simulink model "Algorithm_to_deploy"  (R2025b)
settings: Solver=ode4  StartTime=0.0  StopTime=Tfin  FixedStep=0.005  RelTol=1e-3  EnableMultiTasking=on
undefined symbols (not defined in the file): A_zeta_f, A_zeta_tau, C_zeta_f, C_zeta_tau, eigs_NDO_force, eigs_NDO_torque, F1, F2, inertia_factor, J, m, mass_factor, NDOB_force, NDOB_torque, Ts_hw
settings Model: Creator=baldo  LastModifiedBy=robyd
settings DataIOCC: SaveOutput=off  SaveTime=off
settings OptimizationCC: DefaultParameterBehavior=Inlined  EnhancedBackFolding=on  PassReuseOutputArgsAs=Individual arguments  ZeroExternalMemoryAtStartup=off  ZeroInternalMemoryAtStartup=off  MaxStackSize=512  OptimizeBlockOrder=speed  DifferentSizesBufferReuse=on  OptimizationCustomize=off  EfficientTunableParamExpr=on
settings DebuggingCC: ParameterTunabilityLossMsg=error  UnconnectedInputMsg=warning  UnconnectedOutputMsg=warning  UnconnectedLineMsg=warning
settings HardwareCC: ProdBitPerPointer=32.0  ProdBitPerSizeT=32.0  ProdBitPerPtrDiffT=32.0  ProdLargestAtomicInteger=Long  ProdLargestAtomicFloat=Double  ProdWordSize=32.0  ProdLongLongMode=on  ProdHWDeviceType=ARM Compatible->ARM Cortex-M
settings ModelReferenceCC: EnableRefExpFcnMdlSchedulingChecks=on  PropagateVarSize=During execution
settings SFSimCC: MATLABDynamicMemAlloc=off
settings RTWCC: SystemTargetFile=ert.tlc  HardwareBoard=STM32H7xx Based (Single-core)  TemplateMakefile=ert_default_tmf  Toolchain=GNU Tools for ARM Embedded Processors  CodeExecutionProfiling=on  GPUComputeCapability=3.5  DLArmComputeVersion=19.05  Description=Embedded Coder
settings CodeAppCC: ForceParamTrailComments=on  IgnoreCustomStorageClasses=off  OperatorAnnotations=on  SimulinkDataObjDesc=on  SFDataObjDesc=on  InsertBlockDesc=on
settings ERTTargetCC: ExtModeTransport=3.0  ExtModeStaticAlloc=on  ExtModeStaticAllocSize=2048.0  ExtModeMexFile=ext_xcp  ExtModeIntrfLevel=Level2 - Open  TargetLangStandard=C99 (ISO)  CodeReplacementLibrary=ARM Cortex-M  SupportVariableSizeSignals=on

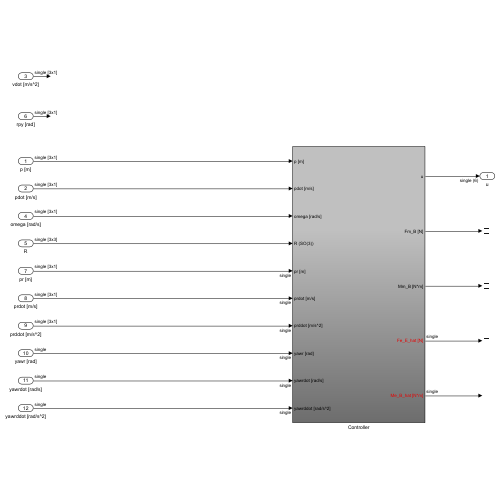
[thumbnail: Simulink's stored preview of the top-level diagram]
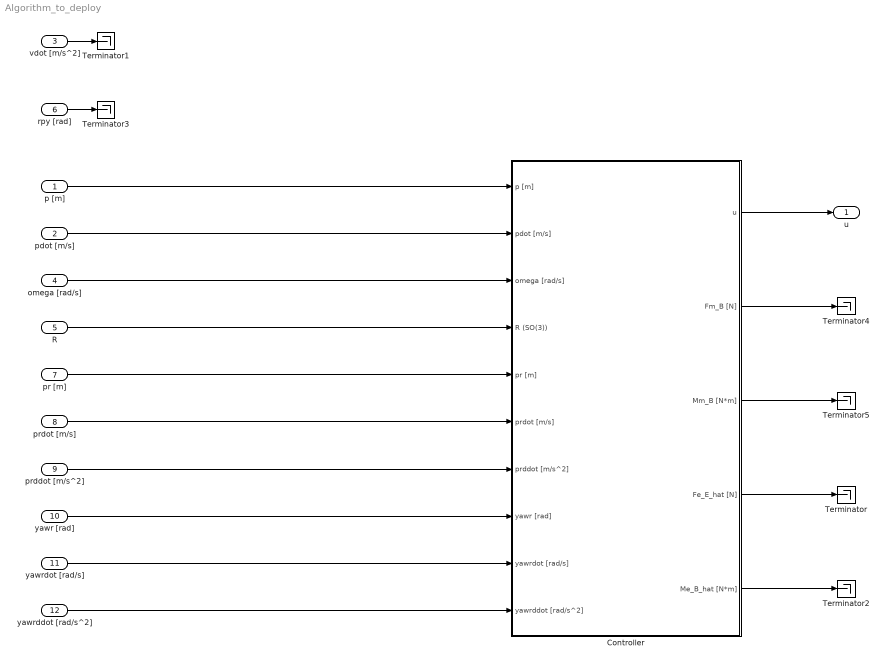
== system Algorithm_to_deploy ==
  p [m] : Inport  OutDataTypeStr=single  PortDimensions=[3 1]  SampleTime=[0.0050000000000000001,0]
  pdot [m/s] : Inport  Port=2  OutDataTypeStr=single  PortDimensions=[3 1]  SampleTime=[0.0050000000000000001,0]
  vdot [m/s^2] : Inport  Port=3  OutDataTypeStr=single  PortDimensions=[3 1]  SampleTime=[0.0050000000000000001,0]
  omega [rad/s] : Inport  Port=4  OutDataTypeStr=single  PortDimensions=[3 1]  SampleTime=[0.0050000000000000001,0]
  R : Inport  Port=5  OutDataTypeStr=single  PortDimensions=[3 3]  SampleTime=[0.0050000000000000001,0]
  rpy [rad] : Inport  Port=6  OutDataTypeStr=single  PortDimensions=[3 1]  SampleTime=[0.0050000000000000001,0]
  pr [m] : Inport  Port=7  OutDataTypeStr=single  PortDimensions=[3 1]  SampleTime=[0.0050000000000000001,0]
  prdot [m/s] : Inport  Port=8  OutDataTypeStr=single  PortDimensions=[3 1]  SampleTime=[0.0050000000000000001,0]
  prddot [m/s^2] : Inport  Port=9  OutDataTypeStr=single  PortDimensions=[3 1]  SampleTime=[0.0050000000000000001,0]
  yawr [rad] : Inport  Port=10  OutDataTypeStr=single  PortDimensions=1  SampleTime=[0.0050000000000000001,0]
  yawrdot [rad/s] : Inport  Port=11  OutDataTypeStr=single  PortDimensions=1  SampleTime=[0.0050000000000000001,0]
  yawrddot [rad/s^2] : Inport  Port=12  OutDataTypeStr=single  PortDimensions=1  SampleTime=[0.0050000000000000001,0]
  Controller : Subsystem
  Terminator{,1..5} (6 alike) : Terminator
  u : Outport  OutDataTypeStr=single  PortDimensions=6  SampleTime=[0.0050000000000000001,0]
  wires:
  vdot [m/s^2]/1 -> Terminator1/1
  rpy [rad]/1 -> Terminator3/1
  p [m]/1 -> Controller/1(p [m])
  pdot [m/s]/1 -> Controller/2(pdot [m/s])
  omega [rad/s]/1 -> Controller/3(omega [rad/s])
  R/1 -> Controller/4(R (SO(3)))
  pr [m]/1 -> Controller/5(pr [m])
  prdot [m/s]/1 -> Controller/6(prdot [m/s])
  prddot [m/s^2]/1 -> Controller/7(prddot [m/s^2])
  yawr [rad]/1 -> Controller/8(yawr [rad])
  yawrdot [rad/s]/1 -> Controller/9(yawrdot [rad/s])
  yawrddot [rad/s^2]/1 -> Controller/10(yawrddot [rad/s^2])
  Controller/1(u) -> u/1
  Controller/2(Fm_B [N]) -> Terminator4/1
  Controller/3(Mm_B [N*m]) -> Terminator5/1
  Controller/4(Fe_E_hat [N]) -> Terminator/1
  Controller/5(Me_B_hat [N*m]) -> Terminator2/1

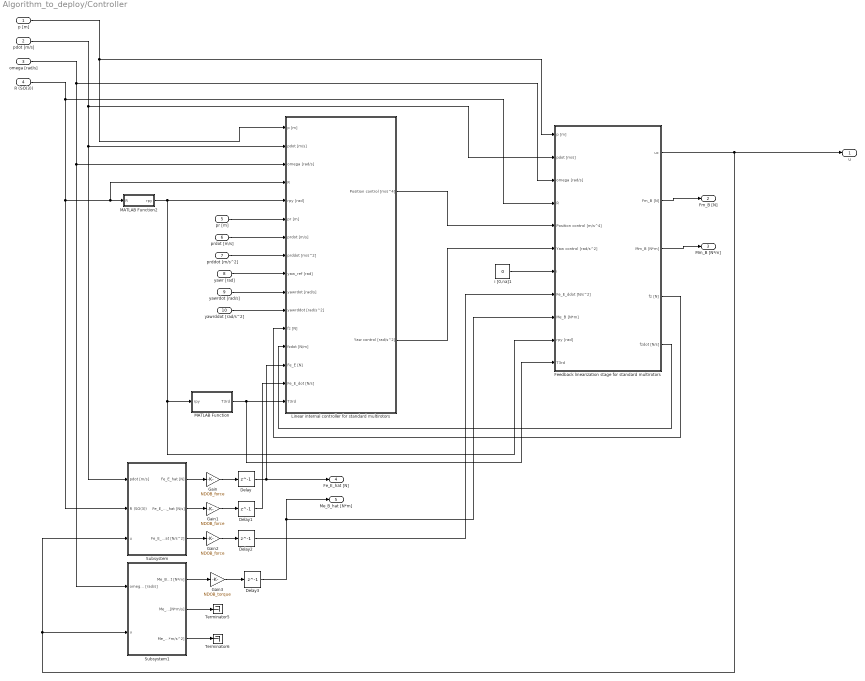
== system Algorithm_to_deploy/Controller ==
  p [m] : Inport
  pdot [m/s] : Inport  Port=2
  omega [rad/s] : Inport  Port=3
  R (SO(3)) : Inport  Port=4
  pr [m] : Inport  Port=5  OutDataTypeStr=single
  prdot [m/s] : Inport  Port=6  OutDataTypeStr=single
  prddot [m/s^2] : Inport  Port=7  OutDataTypeStr=single
  yawr [rad] : Inport  Port=8  OutDataTypeStr=single
  yawrdot [rad/s] : Inport  Port=9  OutDataTypeStr=single
  yawrddot [rad/s^2] : Inport  Port=10  OutDataTypeStr=single
  Delay{,1..3} (4 alike) : Delay  DelayLength=1  InitialCondition=0
  Feedback linearization stage for standard multirotors : Subsystem  mask{mask_m=single(m*mass_factor), mask_J=single(J*inertia_factor), mask_rg_B=zeros(3,1), mask_F1=single(F1), mask_F2=single(F2), mask_thrustmax=1, mask_fz0=single(m*9.8), mask_Ts=Ts_hw}
      mask prompts: mask_m "Mass [kg]"; mask_J "Inertia Tensor [kg*m^2]"; mask_rg_B "Center of mass [m]"; mask_F1 "Control force input matrix"; mask_F2 "Control moment input matrix"; mask_thrustmax "Max thrust [N]"; mask_fz0 "Upward lift force"; mask_Ts "Sample time"
      mask init:
      | % Wrappers
      |     e1 = single([1; 0; 0]);
      |     e2 = single([0; 1; 0]);
      |     e3 = single([0; 0; 1]);
      |     
      |     %%%%%%%%%%%%%%%%%%%%%%%%%%%%%%%%%%%%%%%%%%%%
      |     %    Some general paramater
      |     %%%%%%%%%%%%%%%%%%%%%%%%%%%%%%%%%%%%%%%%%%%%
      |     mask_Jinv = inv(mask_J);
      |     mask_g = single(9.8);
      |     mask_na = size(mask_F1,2);
      | 
      |     %%%%%%%%%%%%%%%%%%%%%%%%%%%%%%%%%%%%%%%%%%%%
      |     %    Allocation for standard multirotors
      |     %%%%%%%%%%%%%%%%%%%%%%%%%%%%%%%%%%%%%%%%%%%%
      |     A = [mask_F1(3,:); mask_F2];
      |     A_pinv = single(pinv(A));
      mask DialogControl DescGroupVar Prompt: Feedback linearization stage for standard multirotors
      mask DialogControl DescTextVar Prompt: Dynamic feedback linearization for standard multirotors. Moore-Penrose allocation. The dynamic estension is "exact".
      mask DialogControl Control3 Prompt: Author: Alessandro Baldini
      mask DialogControl ParameterGroupVar Prompt: Multirotor parameters
      mask DialogControl Container4 Prompt: Initial condition and others
  Gain : Gain  Gain=NDOB_force
  Gain1 : Gain  Gain=NDOB_force
  Gain2 : Gain  Gain=NDOB_force
  Gain3 : Gain  Gain=NDOB_torque
  Linear internal controller for standard multirotors : Subsystem  mask{mask_m=single(m*mass_factor), mask_J=single(J*inertia_factor), mask_rg_B=zeros(3,1), mask_F1=single(F1), mask_F2=single(F2), mask_thrustmax=1, mask_xpoles=single([-3.0 -3.1 -3.2 -3.2 -1.3]/1.3), mask_ypoles=single([-3.0 -3.1 -3.2 -3.2 -1.3]/1.3), mask_zpoles=single([-3.0 -3.1 -3.2 -3.2 -1.3]/1.3), mask_yawpoles=single([-1 -2]), mask_chkPID=off, mask_chkYaw=off, mask_fz0=single(m*9.8), mask_Ts=Ts_hw}
      mask prompts: mask_m "Mass [kg]"; mask_J "Inertia Tensor [kg*m^2]"; mask_rg_B "Center of mass [m]"; mask_F1 "Control force input matrix"; mask_F2 "Control moment input matrix"; mask_thrustmax "Max thrust [N]"; mask_xpoles "Closed loop x poles"; mask_ypoles "Closed loop y poles"; mask_zpoles "Closed loop z poles"; mask_yawpoles "Closed loop yaw poles"; mask_chkPID "Enable position integrators"; mask_chkYaw "Enable yaw integrator"; mask_fz0 "Upward lift force"; mask_Ts "Sample time"
      mask init:
      | % Wrappers
      |     e1 = [1; 0; 0];
      |     e2 = [0; 1; 0];
      |     e3 = [0; 0; 1];
      |     
      |     %%%%%%%%%%%%%%%%%%%%%%%%%%%%%%%%%%%%%%%%%%%%
      |     %    Some general paramater
      |     %%%%%%%%%%%%%%%%%%%%%%%%%%%%%%%%%%%%%%%%%%%%
      |     mask_Jinv = inv(mask_J);
      |     mask_g = 9.8;
      |     mask_na = size(mask_F1,2);
      |     
      |     %%%%%%%%%%%%%%%%%%%%%%%%%%%%%%%%%%%%%%%%%%%%
      |     %    ( Control paramaters)
      |     %%%%%%%%%%%%%%%%%%%%%%%%%%%%%%%%%%%%%%%%%%%%
      |     % Calculation of outer loop parameters
      |     polyx = poly(mask_xpoles);
      |     polyy = poly(mask_ypoles);
      |     polyz = poly(mask_zpoles);
      |     polyyaw = poly(mask_yawpoles);
      | 
      |     if mask_chkPID == 1
      |         % Raw pole placement (with integral action)
      |         % We consider the first 5 poles (2 for yaw)
      |         mask_xpoles = mask_xpoles(1:5);
      |         mask_ypoles = mask_ypoles(1:5);
      |         mask_zpoles = mask_zpoles(1:5);
      |         polyyaw = polyyaw(1:2);
      | 
      |         polyx = poly(mask_xpoles);
      |         polyy = poly(mask_ypoles);
      |         polyz = poly(mask_zpoles);
      |         polyyaw = poly(mask_yawpoles);
      | 
      |         mask_k0 = diag([polyx(6) polyy(6) polyz(6)]);
      |         mask_k1 = diag([polyx(5) polyy(5) polyz(5)]);
      |         mask_k2 = diag([polyx(4) polyy(4) polyz(4)]);
      |         mask_k3 = diag([polyx(3) polyy(3) polyz(3)]);
      |         mask_k4 = diag([polyx(2) polyy(2) polyz(2)]);
      |         
      |         k0yaw = polyyaw(3);
      |         k1yaw = polyyaw(2);
      | 
      |     else
      |         % Raw pole placement (no integral action)
      |         % We consider the first 4 poles (2 for yaw)
      |         mask_xpoles = mask_xpoles(1:4);
      |         mask_ypoles = mask_ypoles(1:4);
      |         mask_zpoles = mask_zpoles(1:4);
      |         polyyaw = polyyaw(1:2);
      | 
      |         polyx = poly(mask_xpoles);
      |         polyy = poly(mask_ypoles);
      |         polyz = poly(mask_zpoles);
      |         polyyaw = poly(mask_yawpoles);
      | 
      |         mask_k0 = diag([polyx(5) polyy(5) polyz(5)]);
      |         mask_k1 = diag([polyx(4) polyy(4) polyz(4)]);
      |         mask_k2 = diag([polyx(3) polyy(3) polyz(3)]);
      |         mask_k3 = diag([polyx(2) polyy(2) polyz(2)]);
      |         mask_k4 = zeros(1,3); % Not used in this control mode
      | 
      |         k0yaw = polyyaw(3);
      |         k1yaw = polyyaw(2);
      |     end
      mask DialogControl DescGroupVar Prompt: Linear controller for standard multirotors
      mask DialogControl DescTextVar Prompt: Linear state space pole placement to couple with a feedback linearization stage. For standard multirotors.
      mask DialogControl Control3 Prompt: Author: Alessandro Baldini
      mask DialogControl ParameterGroupVar Prompt: Multirotor parameters
      mask DialogControl Container3 Prompt: Control paramaters (+1 pole each in case of integrators)
      mask DialogControl Container4 Prompt: Initial condition and others
  MATLAB Function : MATLAB Function  TreatAsAtomicUnit=on
  MATLAB Function2 : MATLAB Function  TreatAsAtomicUnit=on
  Subsystem : Subsystem  mask{mask_m=single(m*mass_factor), mask_F1=single(F1), mask_C=single(C_zeta_f), mask_A=single(A_zeta_f), mask_poles=single(eigs_NDO_force), mask_Ts=Ts_hw}
      mask prompts: mask_m "Mass [kg]"; mask_F1 "Control force input matrix"; mask_C "Exogenous system output matrix C"; mask_A "Exogenous system dynamics matrix A"; mask_poles "Poles to place"; mask_Ts "Sample time"
      mask init:
      | mask_nzeta = size(mask_A,2);
      |     if length(mask_poles) < mask_nzeta
      |         error(num2str(mask_nzeta) + " poles should be specified for the force estimation.")
      |     end
      | 
      |     mask_H = place(mask_A',mask_C',mask_poles(1:mask_nzeta))';
      |     mask_AH = mask_A - mask_H*mask_C;
      |     mask_g = 9.8;
      mask DialogControl DescGroupVar Prompt: Rigid body force observer - v 0.1
      mask DialogControl DescTextVar Prompt: Force observer for a rigid body through a Nonlinear Disturbance Observer (NDO), i.e., reduced order functional observer.
      mask DialogControl Control2 Prompt: Author: Alessandro Baldini
      mask DialogControl Mask_marameters Prompt: Parameters
      mask DialogControl Container3 Prompt: Initial conditions and others
  Subsystem1 : Subsystem  mask{mask_J=single(J*inertia_factor), mask_F2=single(F2), mask_C=single(C_zeta_tau), mask_A=single(A_zeta_tau), mask_poles=single(eigs_NDO_torque), mask_Ts=Ts_hw}
      mask prompts: mask_J "Inertia tensor [kg*m^2]"; mask_F2 "Control moment input matrix"; mask_C "Exogenous system output matrix C"; mask_A "Exogenous system dynamics matrix A"; mask_poles "Poles to place"; mask_Ts "Sample time"
      mask init:
      | mask_nzeta = size(mask_A,2);
      |     if length(mask_poles) < mask_nzeta
      |         error(num2str(mask_nzeta) + " poles should be specified for the torque estimation.")
      |     end
      | 
      |     mask_H = place(mask_A',mask_C',mask_poles(1:mask_nzeta))';
      |     mask_AH = mask_A - mask_H*mask_C;
      mask DialogControl DescGroupVar Prompt: Rigid body torque observer - v 0.1
      mask DialogControl DescTextVar Prompt: Torque observer for a rigid body through a Nonlinear Disturbance Observer (NDO), i.e., reduced order functional observer.
      mask DialogControl Control2 Prompt: Author: Alessandro Baldini
      mask DialogControl Mask_marameters Prompt: Parameters
      mask DialogControl Container3 Prompt: Initial conditions and others
  Terminator5 : Terminator
  Terminator6 : Terminator
  i [0,na]1 : Constant  Value=0  OutDataTypeStr=single  SampleTime=Ts_hw
  u : Outport
  Fm_B [N] : Outport  Port=2
  Mm_B [N*m] : Outport  Port=3
  Fe_E_hat [N] : Outport  Port=4  OutDataTypeStr=single
  Me_B_hat [N*m] : Outport  Port=5  OutDataTypeStr=single
  wires:
  i [0,na]1/1 -> Feedback linearization stage for standard multirotors/7(i)
  Gain3/1 -> Delay3/1
  Delay3/1 -> Feedback linearization stage for standard multirotors/9(Me_B [N*m]), Me_B_hat [N*m]/1
  Gain2/1 -> Delay2/1
  Subsystem1/2(Me_B_dot_hat [N*m/s]) -> Terminator5/1
  Feedback linearization stage for standard multirotors/3(Mm_B [N*m]) -> Mm_B [N*m]/1
  prddot [m/s^2]/1 -> Linear internal controller for standard multirotors/8(prddot [m/s^2])
  p [m]/1 -> Feedback linearization stage for standard multirotors/1(p [m]), Linear internal controller for standard multirotors/1(p [m])
  yawrddot [rad/s^2]/1 -> Linear internal controller for standard multirotors/11(yawrddot [rad/s^2])
  yawrdot [rad/s]/1 -> Linear internal controller for standard multirotors/10(yawrdot [rad/s])
  omega [rad/s]/1 -> Feedback linearization stage for standard multirotors/3(omega [rad/s]), Linear internal controller for standard multirotors/3(omega [rad/s]), Subsystem1/1(omega [rad/s])
  Subsystem1/1(Me_B_hat [N*m]) -> Gain3/1
  Linear internal controller for standard multirotors/1(" Position control [m/s^4]") -> Feedback linearization stage for standard multirotors/5(Position control [m/s^4])
  Gain1/1 -> Delay1/1
  Subsystem/1(Fe_E_hat [N]) -> Gain/1
  Subsystem/2(Fe_E_dot_hat [N/s]) -> Gain1/1
  Feedback linearization stage for standard multirotors/1(uc) -> Subsystem1/2(u), Subsystem/3(u), u/1
  Subsystem/3(Fe_E_ddot_hat [N/s^2]) -> Gain2/1
  Subsystem1/3(Me_B_ddot_hat [N*m/s^2]) -> Terminator6/1
  R (SO(3))/1 -> Subsystem/2(R (SO(3))), MATLAB Function2/1(R), Linear internal controller for standard multirotors/4(R), Feedback linearization stage for standard multirotors/4(R)
  Feedback linearization stage for standard multirotors/4(fz [N]) -> Linear internal controller for standard multirotors/12(fz [N])
  Feedback linearization stage for standard multirotors/5(fzdot [N/s]) -> Linear internal controller for standard multirotors/13(fzdot [N/m])
  prdot [m/s]/1 -> Linear internal controller for standard multirotors/7(prdot [m/s])
  Gain/1 -> Delay/1
  MATLAB Function2/1(rpy) -> MATLAB Function/1(rpy), Feedback linearization stage for standard multirotors/10(rpy [rad]), Linear internal controller for standard multirotors/5(rpy [rad])
  yawr [rad]/1 -> Linear internal controller for standard multirotors/9(yaw_ref [rad])
  Delay1/1 -> Linear internal controller for standard multirotors/15(Fe_E_dot [N/s])
  MATLAB Function/1(T3rd) -> Linear internal controller for standard multirotors/16(T3rd), Feedback linearization stage for standard multirotors/11(T3rd)
  Delay/1 -> Linear internal controller for standard multirotors/14(Fe_E [N]), Fe_E_hat [N]/1
  Delay2/1 -> Feedback linearization stage for standard multirotors/8(Fe_E_ddot [N/s^2])
  pdot [m/s]/1 -> Linear internal controller for standard multirotors/2(pdot [m/s]), Subsystem/1(pdot [m/s]), Feedback linearization stage for standard multirotors/2(pdot [m/s])
  Linear internal controller for standard multirotors/2(" Yaw control [rad/s^2]") -> Feedback linearization stage for standard multirotors/6(Yaw control [rad/s^2])
  pr [m]/1 -> Linear internal controller for standard multirotors/6(pr [m])
  Feedback linearization stage for standard multirotors/2(Fm_B [N]) -> Fm_B [N]/1

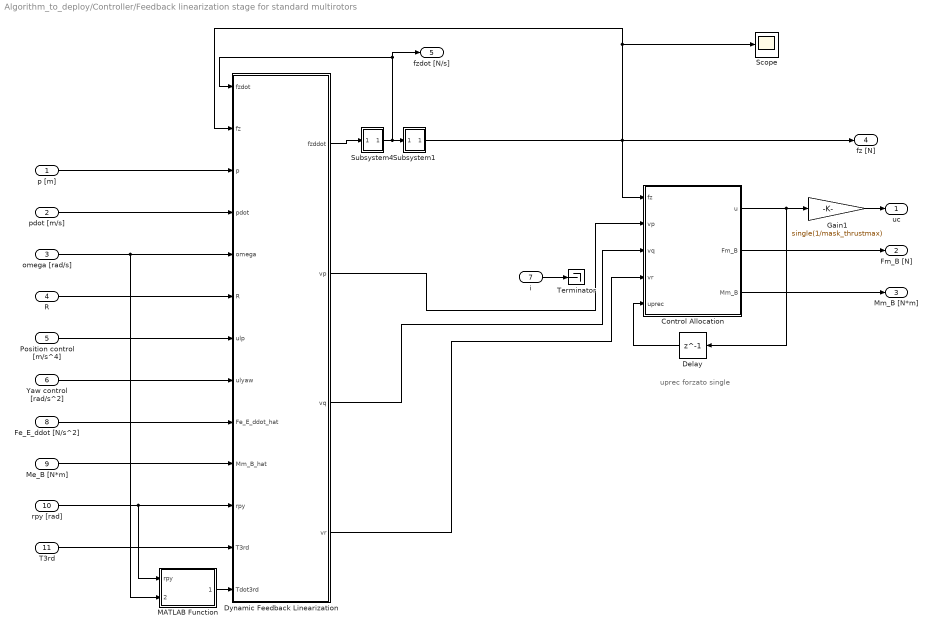
== system Algorithm_to_deploy/Controller/Feedback linearization stage for standard multirotors ==
  note: uprec forzato single
  p [m] : Inport
  pdot [m/s] : Inport  Port=2
  omega [rad/s] : Inport  Port=3
  R : Inport  Port=4
  Position control [m/s^4] : Inport  Port=5
  Yaw control [rad/s^2] : Inport  Port=6
  i : Inport  Port=7
  Fe_E_ddot [N/s^2] : Inport  Port=8
  Me_B [N*m] : Inport  Port=9
  rpy [rad] : Inport  Port=10
  T3rd : Inport  Port=11
  Control Allocation : MATLAB Function  TreatAsAtomicUnit=on
  Delay : Delay  DelayLength=1  InitialCondition=0
  Dynamic Feedback Linearization : MATLAB Function  TreatAsAtomicUnit=on
  Gain1 : Gain  Gain=single(1/mask_thrustmax)
  MATLAB Function : MATLAB Function  TreatAsAtomicUnit=on
  Scope : Scope
      settings: ActiveDisplayYMinimum=13.64532  ActiveDisplayYMaximum=29.09214
  Subsystem1 : Subsystem  mask{mask_IC=single(mask_m*mask_g), mask_ts=mask_Ts}
      mask prompts: mask_IC "Initial condition"; mask_ts "Sample time"
      mask DialogControl DescGroupVar Prompt: Backward Euler integrator
      mask DialogControl DescTextVar Prompt: Discrete time block approximating an integrator through backward Euler.
  Subsystem4 : Subsystem  mask{mask_IC=single(zeros(1,1)), mask_ts=mask_Ts}
      mask prompts: mask_IC "Initial condition"; mask_ts "Sample time"
      mask DialogControl DescGroupVar Prompt: Backward Euler integrator
      mask DialogControl DescTextVar Prompt: Discrete time block approximating an integrator through backward Euler.
  Terminator : Terminator
  uc : Outport  PortDimensions=mask_na
  Fm_B [N] : Outport  Port=2  PortDimensions=3
  Mm_B [N*m] : Outport  Port=3  PortDimensions=3
  fz [N] : Outport  Port=4
  fzdot [N/s] : Outport  Port=5
  wires:
  MATLAB Function/1(Tdot3rd) -> Dynamic Feedback Linearization/13(Tdot3rd)
  T3rd/1 -> Dynamic Feedback Linearization/12(T3rd)
  rpy [rad]/1 -> MATLAB Function/1(rpy), Dynamic Feedback Linearization/11(rpy)
  i/1 -> Terminator/1
  Fe_E_ddot [N/s^2]/1 -> Dynamic Feedback Linearization/9(Fe_E_ddot_hat)
  Me_B [N*m]/1 -> Dynamic Feedback Linearization/10(Mm_B_hat)
  Yaw control [rad/s^2]/1 -> Dynamic Feedback Linearization/8(ulyaw)
  Position control [m/s^4]/1 -> Dynamic Feedback Linearization/7(ulp)
  Gain1/1 -> uc/1
  Control Allocation/2(Fm_B) -> Fm_B [N]/1
  Control Allocation/1(u) -> Delay/1, Gain1/1
  Control Allocation/3(Mm_B) -> Mm_B [N*m]/1
  Delay/1 -> Control Allocation/5(uprec)
  Dynamic Feedback Linearization/4(vr) -> Control Allocation/4(vr)
  Dynamic Feedback Linearization/2(vp) -> Control Allocation/2(vp)
  Subsystem1/1(Out1) -> Control Allocation/1(fz), fz [N]/1, Scope/1, Dynamic Feedback Linearization/2(fz)
  Dynamic Feedback Linearization/3(vq) -> Control Allocation/3(vq)
  Subsystem4/1(Out1) -> Dynamic Feedback Linearization/1(fzdot), fzdot [N/s]/1, Subsystem1/1(In1)
  Dynamic Feedback Linearization/1(fzddot) -> Subsystem4/1(In1)
  p [m]/1 -> Dynamic Feedback Linearization/3(p)
  R/1 -> Dynamic Feedback Linearization/6(R)
  pdot [m/s]/1 -> Dynamic Feedback Linearization/4(pdot)
  omega [rad/s]/1 -> Dynamic Feedback Linearization/5(omega), MATLAB Function/2(omega)

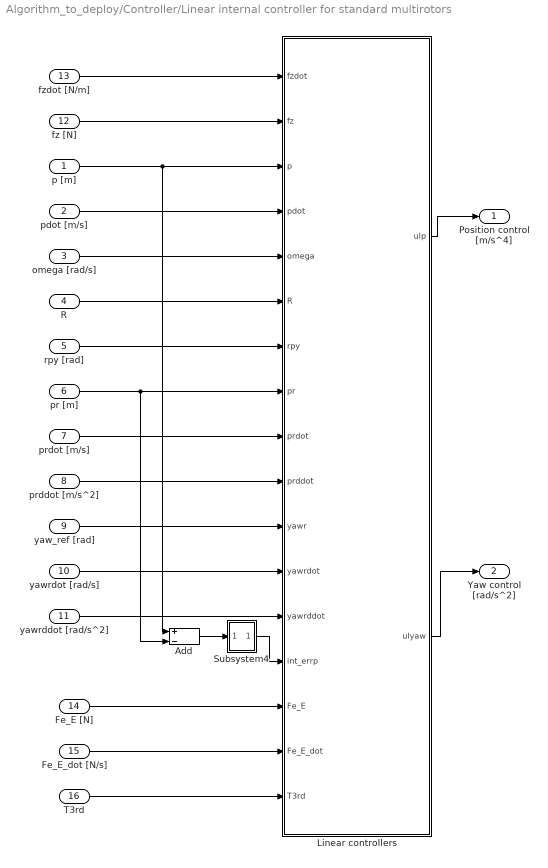
== system Algorithm_to_deploy/Controller/Linear internal controller for standard multirotors ==
  p [m] : Inport
  pdot [m/s] : Inport  Port=2
  omega [rad/s] : Inport  Port=3
  R : Inport  Port=4
  rpy [rad] : Inport  Port=5
  pr [m] : Inport  Port=6
  prdot [m/s] : Inport  Port=7
  prddot [m/s^2] : Inport  Port=8
  yaw_ref [rad] : Inport  Port=9
  yawrdot [rad/s] : Inport  Port=10
  yawrddot [rad/s^2] : Inport  Port=11
  fz [N] : Inport  Port=12
  fzdot [N/m] : Inport  Port=13
  Fe_E [N] : Inport  Port=14
  Fe_E_dot [N/s] : Inport  Port=15
  T3rd : Inport  Port=16
  Add : Sum  Inputs=+-
  Linear controllers : MATLAB Function  TreatAsAtomicUnit=on
  Subsystem4 : Subsystem  mask{mask_IC=single(zeros(1,1)), mask_ts=mask_Ts}
      mask prompts: mask_IC "Initial condition"; mask_ts "Sample time"
      mask DialogControl DescGroupVar Prompt: Backward Euler integrator
      mask DialogControl DescTextVar Prompt: Discrete time block approximating an integrator through backward Euler.
  " Position control [m/s^4]" : Outport
  " Yaw control [rad/s^2]" : Outport  Port=2
  wires:
  T3rd/1 -> Linear controllers/17(T3rd)
  Fe_E [N]/1 -> Linear controllers/15(Fe_E)
  Fe_E_dot [N/s]/1 -> Linear controllers/16(Fe_E_dot)
  rpy [rad]/1 -> Linear controllers/7(rpy)
  fz [N]/1 -> Linear controllers/2(fz)
  fzdot [N/m]/1 -> Linear controllers/1(fzdot)
  Linear controllers/2(ulyaw) -> " Yaw control [rad/s^2]"/1
  Linear controllers/1(ulp) -> " Position control [m/s^4]"/1
  Subsystem4/1(Out1) -> Linear controllers/14(int_errp)
  Add/1 -> Subsystem4/1(In1)
  yawrddot [rad/s^2]/1 -> Linear controllers/13(yawrddot)
  yawrdot [rad/s]/1 -> Linear controllers/12(yawrdot)
  yaw_ref [rad]/1 -> Linear controllers/11(yawr)
  prdot [m/s]/1 -> Linear controllers/9(prdot)
  prddot [m/s^2]/1 -> Linear controllers/10(prddot)
  p [m]/1 -> Linear controllers/3(p), Add/1
  R/1 -> Linear controllers/6(R)
  pdot [m/s]/1 -> Linear controllers/4(pdot)
  pr [m]/1 -> Linear controllers/8(pr), Add/2
  omega [rad/s]/1 -> Linear controllers/5(omega)

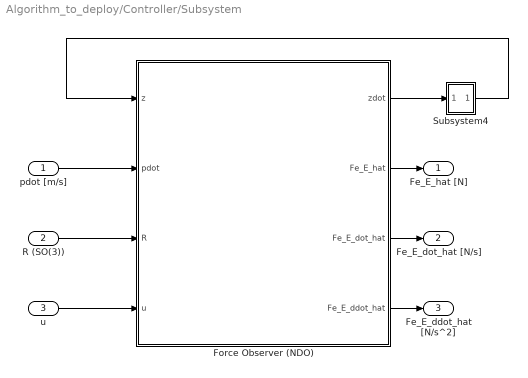
== system Algorithm_to_deploy/Controller/Subsystem ==
  pdot [m/s] : Inport
  R (SO(3)) : Inport  Port=2
  u : Inport  Port=3
  Force Observer (NDO) : MATLAB Function  TreatAsAtomicUnit=on
  Subsystem4 : Subsystem  mask{mask_IC=single(zeros(mask_nzeta,1)), mask_ts=mask_Ts}
      mask prompts: mask_IC "Initial condition"; mask_ts "Sample time"
      mask DialogControl DescGroupVar Prompt: Backward Euler integrator
      mask DialogControl DescTextVar Prompt: Discrete time block approximating an integrator through backward Euler.
  Fe_E_hat [N] : Outport
  Fe_E_dot_hat [N/s] : Outport  Port=2
  Fe_E_ddot_hat [N/s^2] : Outport  Port=3
  wires:
  R (SO(3))/1 -> Force Observer (NDO)/3(R)
  pdot [m/s]/1 -> Force Observer (NDO)/2(pdot)
  Force Observer (NDO)/4(Fe_E_ddot_hat) -> Fe_E_ddot_hat [N/s^2]/1
  u/1 -> Force Observer (NDO)/4(u)
  Force Observer (NDO)/2(Fe_E_hat) -> Fe_E_hat [N]/1
  Subsystem4/1(Out1) -> Force Observer (NDO)/1(z)
  Force Observer (NDO)/3(Fe_E_dot_hat) -> Fe_E_dot_hat [N/s]/1
  Force Observer (NDO)/1(zdot) -> Subsystem4/1(In1)

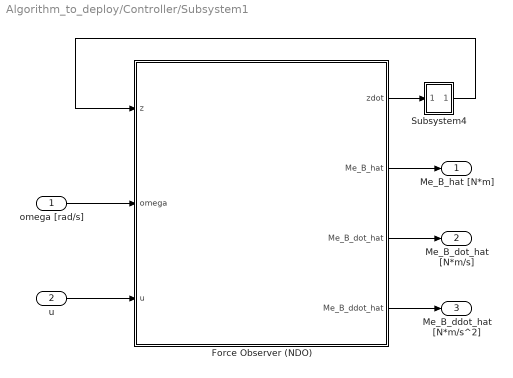
== system Algorithm_to_deploy/Controller/Subsystem1 ==
  omega [rad/s] : Inport
  u : Inport  Port=2
  Force Observer (NDO) : MATLAB Function  TreatAsAtomicUnit=on
  Subsystem4 : Subsystem  mask{mask_IC=single(zeros(mask_nzeta,1)), mask_ts=mask_Ts}
      mask prompts: mask_IC "Initial condition"; mask_ts "Sample time"
      mask DialogControl DescGroupVar Prompt: Backward Euler integrator
      mask DialogControl DescTextVar Prompt: Discrete time block approximating an integrator through backward Euler.
  Me_B_hat [N*m] : Outport
  Me_B_dot_hat [N*m/s] : Outport  Port=2
  Me_B_ddot_hat [N*m/s^2] : Outport  Port=3
  wires:
  Force Observer (NDO)/1(zdot) -> Subsystem4/1(In1)
  Force Observer (NDO)/3(Me_B_dot_hat) -> Me_B_dot_hat [N*m/s]/1
  Subsystem4/1(Out1) -> Force Observer (NDO)/1(z)
  Force Observer (NDO)/2(Me_B_hat) -> Me_B_hat [N*m]/1
  u/1 -> Force Observer (NDO)/3(u)
  Force Observer (NDO)/4(Me_B_ddot_hat) -> Me_B_ddot_hat [N*m/s^2]/1
  omega [rad/s]/1 -> Force Observer (NDO)/2(omega)

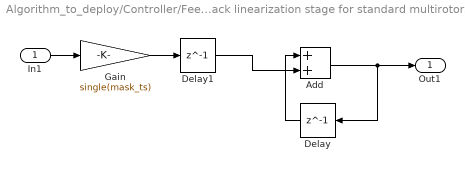
== system Algorithm_to_deploy/Controller/Feedback linearization stage for standard multirotors/Subsystem1 ==
  In1 : Inport
  Add : Sum  OutDataTypeStr=single
  Delay : Delay  DelayLength=1  InitialCondition=mask_IC
  Delay1 : Delay  DelayLength=1  InitialCondition=0*mask_IC
  Gain : Gain  Gain=single(mask_ts)
  Out1 : Outport
  wires:
  Add/1 -> Out1/1, Delay/1
  Gain/1 -> Delay1/1
  In1/1 -> Gain/1
  Delay1/1 -> Add/2
  Delay/1 -> Add/1

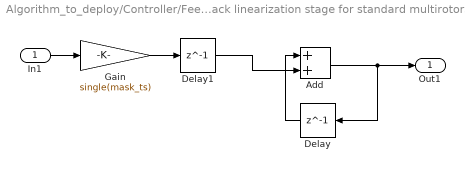
== system Algorithm_to_deploy/Controller/Feedback linearization stage for standard multirotors/Subsystem4 ==
  In1 : Inport
  Add : Sum  OutDataTypeStr=single
  Delay : Delay  DelayLength=1  InitialCondition=mask_IC
  Delay1 : Delay  DelayLength=1  InitialCondition=0*mask_IC
  Gain : Gain  Gain=single(mask_ts)
  Out1 : Outport
  wires:
  Delay/1 -> Add/1
  Delay1/1 -> Add/2
  In1/1 -> Gain/1
  Gain/1 -> Delay1/1
  Add/1 -> Delay/1, Out1/1

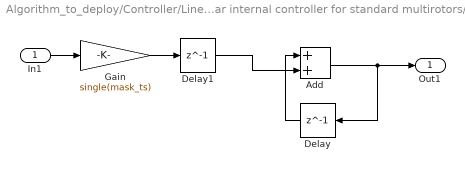
== system Algorithm_to_deploy/Controller/Linear internal controller for standard multirotors/Subsystem4 ==
  In1 : Inport
  Add : Sum  OutDataTypeStr=single
  Delay : Delay  DelayLength=1  InitialCondition=mask_IC
  Delay1 : Delay  DelayLength=1  InitialCondition=0*mask_IC
  Gain : Gain  Gain=single(mask_ts)
  Out1 : Outport
  wires:
  Delay/1 -> Add/1
  Delay1/1 -> Add/2
  In1/1 -> Gain/1
  Gain/1 -> Delay1/1
  Add/1 -> Delay/1, Out1/1

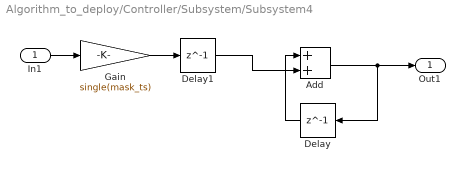
== system Algorithm_to_deploy/Controller/Subsystem/Subsystem4 ==
  In1 : Inport
  Add : Sum  OutDataTypeStr=single
  Delay : Delay  DelayLength=1  InitialCondition=mask_IC
  Delay1 : Delay  DelayLength=1  InitialCondition=0*mask_IC
  Gain : Gain  Gain=single(mask_ts)
  Out1 : Outport
  wires:
  Delay/1 -> Add/1
  Delay1/1 -> Add/2
  In1/1 -> Gain/1
  Gain/1 -> Delay1/1
  Add/1 -> Delay/1, Out1/1

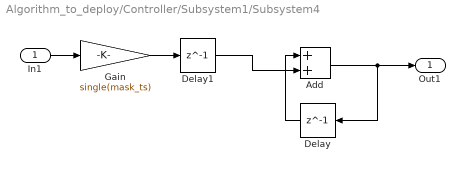
== system Algorithm_to_deploy/Controller/Subsystem1/Subsystem4 ==
  In1 : Inport
  Add : Sum  OutDataTypeStr=single
  Delay : Delay  DelayLength=1  InitialCondition=mask_IC
  Delay1 : Delay  DelayLength=1  InitialCondition=0*mask_IC
  Gain : Gain  Gain=single(mask_ts)
  Out1 : Outport
  wires:
  Add/1 -> Out1/1, Delay/1
  Gain/1 -> Delay1/1
  In1/1 -> Gain/1
  Delay1/1 -> Add/2
  Delay/1 -> Add/1

== matlab function Algorithm_to_deploy/Controller/Feedback linearization stage for standard multirotors/Control Allocation ==
  data: fz input; vp input; vq input; vr input; u output; uprec input single; mask_J parameter; A_pinv parameter; Fm_B output; Mm_B output; mask_na parameter
function [u,Fm_B,Mm_B] = ControlAllocation(fz,vp,vq,vr,uprec, mask_J,A_pinv,mask_na)

Fm_B = [0; 0; -fz];
Mm_B = mask_J*[vp; vq; vr];
b = [-fz; Mm_B];

% Calculation of forces
u = A_pinv*b;

end

== matlab function Algorithm_to_deploy/Controller/Subsystem/Force Observer (NDO) ==
  data: z input; pdot input; R input; u input; zdot output; Fe_E_hat output; Fe_E_dot_hat output; Fe_E_ddot_hat output; mask_F1 parameter; mask_g parameter; mask_m parameter; mask_C parameter; mask_A parameter; mask_AH parameter; mask_H parameter
function [zdot,Fe_E_hat,Fe_E_dot_hat,Fe_E_ddot_hat] = ForceNDO(z,pdot,R,u,mask_F1, mask_g, mask_m, mask_C, mask_A, mask_AH,mask_H)

% Constants
e3 = [0; 0; 1];

zetahat = z + mask_H*mask_m*pdot;
zdot = mask_AH*zetahat - mask_H*(mask_m*mask_g*e3 + R*mask_F1*u);
Fe_E_hat = mask_C*zetahat;
Fe_E_dot_hat = mask_C*mask_A*zetahat;
Fe_E_ddot_hat = mask_C*mask_A^2*zetahat;

end

== matlab function Algorithm_to_deploy/Controller/Feedback linearization stage for standard multirotors/Dynamic Feedback Linearization ==
  data: fzdot input; fzddot output; fz input; p input; pdot input; omega input; R input; ulp input; ulyaw input; vp output; mask_m parameter; mask_g parameter; Fe_E_ddot_hat input; Mm_B_hat input; mask_Jinv parameter; mask_J parameter; vq output; vr output; mask_na parameter; rpy input; T3rd input; Tdot3rd input
function [fzddot,vp,vq,vr] = Control(fzdot,fz,p,pdot,omega,R,ulp,ulyaw,mask_m, mask_g,Fe_E_ddot_hat,Mm_B_hat,mask_Jinv, mask_J,mask_na, rpy,T3rd,Tdot3rd)

% Constants
e1 = [1; 0; 0];
e2 = [0; 1; 0];
e3 = [0; 0; 1];

% Wrappers for short code
m = mask_m;
g = mask_g;
J = mask_J;
Jinv = mask_Jinv;

% General Kinematics
omegae = R*omega;
zB = R*e3;
zBdot = cross(omegae,zB);

% Lie derivatives
gomega = -Jinv*cross(omega,J*omega);
ge = R*gomega;
gp = -2*fzdot*zBdot - fz*(cross(omegae,zBdot) + cross(ge,zB));

% Linearization actions
out = R'*(-gp - fz*cross(zB,R*Jinv*Mm_B_hat) - Fe_E_ddot_hat + m*ulp);
fzddot = -out(3);
vp = out(2)/fz;
vq = -out(1)/fz;

% % Small angle approximation
% vr = -(e3'*gomega) + ulyaw;

% No small angle approximation
vr = (-Tdot3rd*omega - T3rd*gomega - T3rd(1)*vp - T3rd(2)*vq - T3rd*Jinv*Mm_B_hat + ulyaw)/T3rd(3);

% CONTROL - Constant Yaw v1
if norm(fz)<1e-3
    fz = 1e-3;
    error('Upward lift force can not be null. Singular point.')
end

end


function vhat = skew(v)
    e1 = [1 0 0]';
    e2 = [0 1 0]';
    e3 = [0 0 1]';
    vhat = [cross(v,e1) cross(v,e2) cross(v,e3)];
end

== matlab function Algorithm_to_deploy/Controller/Subsystem1/Force Observer (NDO) ==
  data: z input; omega input; u input; zdot output; Me_B_hat output; Me_B_dot_hat output; Me_B_ddot_hat output; mask_J parameter; mask_C parameter; mask_A parameter; mask_AH parameter; mask_H parameter; mask_F2 parameter
function [zdot,Me_B_hat,Me_B_dot_hat,Me_B_ddot_hat] = TorqueNDO(z,omega,u,mask_J, mask_C, mask_A, mask_AH,mask_H, mask_F2)

zetahat = z + mask_H*mask_J*omega;
zdot = mask_AH*zetahat - mask_H*(-cross(omega,mask_J*omega) + mask_F2*u);
Me_B_hat = mask_C*zetahat;
Me_B_dot_hat = mask_C*mask_A*zetahat;
Me_B_ddot_hat = mask_C*mask_A^2*zetahat;

end

== matlab function Algorithm_to_deploy/Controller/MATLAB Function2 ==
  data: R input; rpy output
function rpy = fcn(R)

[rpy_new,~] = rotm2eul(R);
rpy = flip(rpy_new');

end

== matlab function Algorithm_to_deploy/Controller/Feedback linearization stage for standard multirotors/MATLAB Function ==
  data: rpy input; Tdot3rd output; omega input
function Tdot3rd = getTdot(rpy,omega)
    % Calculate the time derivative of the kinematic coordinate tranformation
    % related to roll-pitch-yaw angles
    % T = getT(eta,omega), where eta = [phi; theta; psi] and omega = [p; q; r]
    % T = getT(phi,theta,psi,p,q,r)
    %
    % phi, theta, psi are, in order, roll, pitch and yaw angles.
    phi = rpy(1);
    theta = rpy(2);
    p = omega(1);
    q = omega(2);
    r = omega(3);
    Tdot3rd = [0,(cos(phi)*(p + r*cos(phi)*tan(theta) + q*sin(phi)*tan(theta)))/cos(theta) + (sin(phi)*sin(theta)*(q*cos(phi) - r*sin(phi)))/cos(theta)^2,(cos(phi)*sin(theta)*(q*cos(phi) - r*sin(phi)))/cos(theta)^2 - (sin(phi)*(p + r*cos(phi)*tan(theta) + q*sin(phi)*tan(theta)))/cos(theta)];
end

== matlab function Algorithm_to_deploy/Controller/MATLAB Function ==
  data: rpy input; T3rd output
function T3rd = getT(rpy)
    phi = rpy(1);
    theta = rpy(2);
    
    T3rd = [0 sin(phi)/cos(theta) cos(phi)/cos(theta)];
end

== matlab function Algorithm_to_deploy/Controller/Linear internal controller for standard multirotors/Linear controllers ==
  data: fzdot input; ulp output; fz input; p input; pdot input; omega input; R input; rpy input; pr input; prdot input; prddot input; yawr input; yawrdot input; yawrddot input; int_errp input; ulyaw output; mask_m parameter; mask_g parameter; mask_k0 parameter; mask_k1 parameter; mask_k2 parameter; mask_k3 parameter; mask_k4 parameter; mask_chkPID parameter; Fe_E input; Fe_E_dot input; T3rd input
function [ulp,ulyaw] = LinearControl(fzdot,fz,p,pdot,omega,R,rpy,pr,prdot,prddot,yawr,yawrdot,yawrddot,int_errp,mask_m, mask_g,mask_k0, mask_k1, mask_k2, mask_k3, mask_k4,mask_chkPID,Fe_E,Fe_E_dot,T3rd)

% Constants
e1 = [1; 0; 0];
e2 = [0; 1; 0];
e3 = [0; 0; 1];

% Wrappers for short code
m = mask_m;
g = mask_g;
k0 = mask_k0;
k1 = mask_k1;
k2 = mask_k2;
k3 = mask_k3;
k4 = mask_k4;

% General Kinematics
omegae = R*omega;
zB = R*e3;
zBdot = cross(omegae,zB);

% %%%%%%%%%%%%%%%%%%%%%%%%%%%%%%%%%%%%%%%%%%%%%
% %       Linear position controller #1       %
% %%%%%%%%%%%%%%%%%%%%%%%%%%%%%%%%%%%%%%%%%%%%%
% Linear motion
prddddot = zeros(3,1);
prdddot = zeros(3,1);
pddot = (m*g*e3-fz*zB + Fe_E)/m;
pdddot = (-fzdot*zB-fz*zBdot + Fe_E_dot)/m;
if mask_chkPID == 1
    ulp = prddddot - k4*(pdddot-prdddot) - k3*(pddot-prddot) - k2*(pdot-prdot) - k1*(p-pr) - k0*int_errp;
else
    ulp = prddddot - k3*(pdddot-prdddot) - k2*(pddot-prddot) - k1*(pdot-prdot) - k0*(p-pr);
end

% %%%%%%%%%%%%%%%%%%%%%%%%%%%%%%%%%%%%%%%%%%%%%
% %          Linear yaw controller #1         %
% %%%%%%%%%%%%%%%%%%%%%%%%%%%%%%%%%%%%%%%%%%%%%
polyyaw = poly([-1 -2]);
k0yaw = polyyaw(3);
k1yaw = polyyaw(2);
yaw = rpy(3);

% Small angle approzimation
% ulyaw = + yawrddot - k1yaw*(e3'*omega-yawrdot) - k0yaw*(yaw-yawr);   

% No small angle approximation
ulyaw = + yawrddot - k1yaw*(T3rd*omega-yawrdot) - k0yaw*(yaw-yawr);

end
